simulink model "Subsystem"  (R2020b)
settings: Solver=VariableStepAuto  StartTime=0.0  StopTime=50  RelTol=1e-3
settings Model: Creator=baner  LastModifiedBy=baner
settings DataIOCC: SaveOutput=off  SaveTime=off

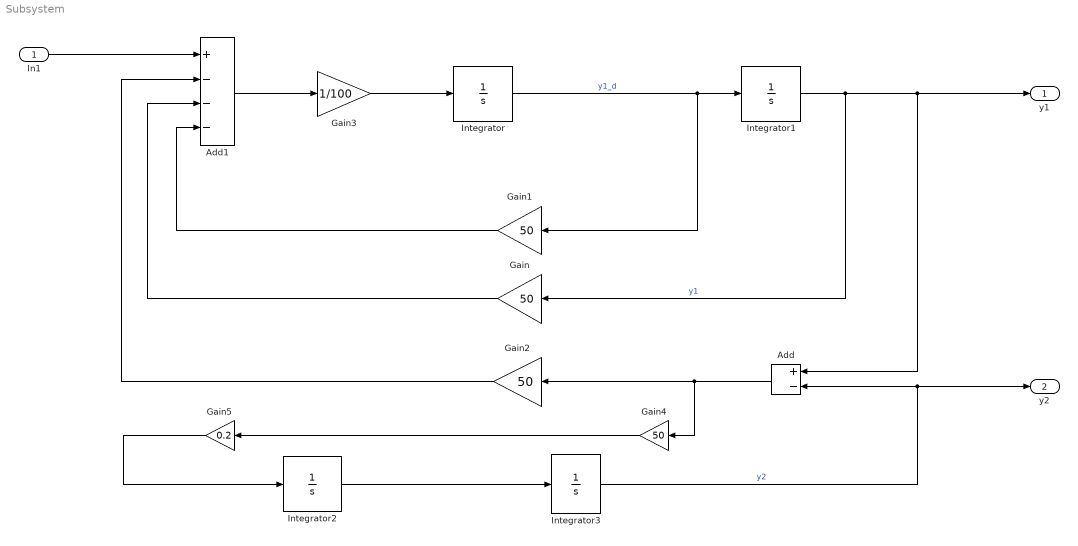
== system Subsystem ==
  In1 : Inport  OutDataTypeStr=double  PortDimensions=1  SampleTime=0
  Add : Sum  Inputs=+-
  Add1 : Sum  Inputs=+---
  Gain{,1..2,4} (4 alike) : Gain  Gain=50
  Gain3 : Gain  Gain=1/100
  Gain5 : Gain  Gain=0.2
  Integrator{,1..3} (4 alike) : Integrator
  y1 : Outport  OutDataTypeStr=double  PortDimensions=1  SampleTime=0
  y2 : Outport  Port=2  OutDataTypeStr=double  PortDimensions=1  SampleTime=0
  wires:
  In1/1 -> Add1/1
  Integrator/1 -> Integrator1/1, Gain1/1  "y1_d"
  Gain2/1 -> Add1/2
  Gain/1 -> Add1/3
  Integrator1/1 -> Gain/1, Add/1, y1/1  "y1"
  Gain3/1 -> Integrator/1
  Integrator3/1 -> Add/2, y2/1  "y2"
  Add1/1 -> Gain3/1
  Integrator2/1 -> Integrator3/1
  Gain1/1 -> Add1/4
  Add/1 -> Gain2/1, Gain4/1
  Gain4/1 -> Gain5/1
  Gain5/1 -> Integrator2/1
